simulink model "__AAVAvionics"  (Simulink 6.0)
settings: Solver=ode45  StartTime=0.0  StopTime=10.0  RelTol=1e-3
settings Model: LastModifiedBy=root

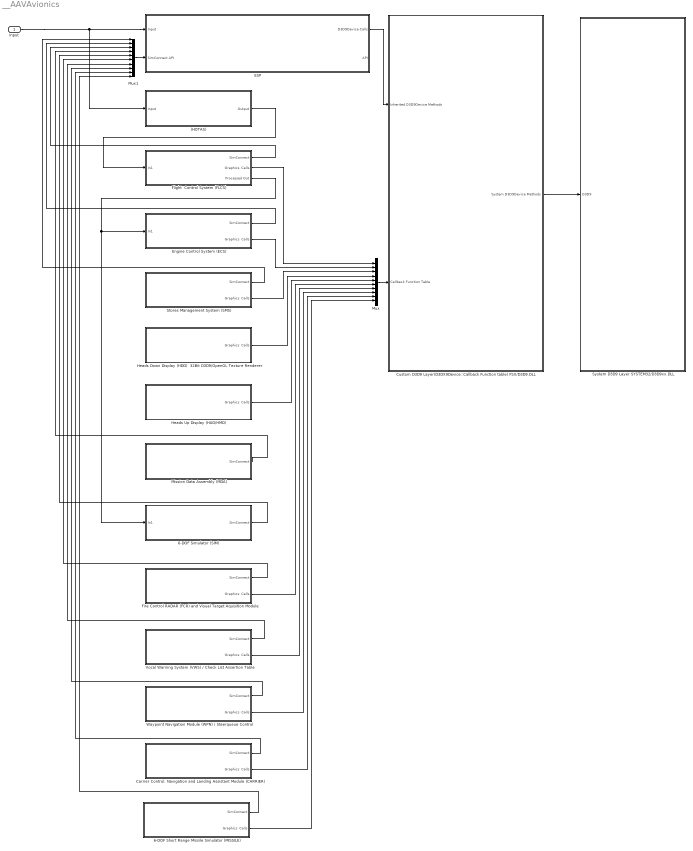
== system __AAVAvionics ==
  Input : Inport  Port=1  LatchInput=off
  (HOTAS) : Subsystem
  6-DOF Short Range Missile Simulator (MISSILE) : Subsystem
  6-DOF Simulator (SIM) : Subsystem
  "Carrier Control, Navigation and Landing Assistant Module (CARRIER)" : Subsystem
  Custom D3D9 Layer(D3DX9Device::Callback Function table) FSX/D3D9.DLL : Subsystem
  ESP : Subsystem
  Engine Control System (ECS) : Subsystem
  Fire Control RADAR (FCR) and Visual Target Aquisition Module : Subsystem
  Flight  Control System (FLCS) : Subsystem
  Heads Down Display (HDD)  32Bit D3D9/OpenGL Texture Renderer : Subsystem
  Heads Up Display (HUD/HMD) : Subsystem
  Mission Data Assembly (MDA) : Subsystem
  Mux : Mux  Inputs=10
  Mux1 : Mux  Inputs=10
  Stores Management System (SMS) : Subsystem
  System D3D9 Layer SYSTEM32/D3D9xx.DLL : Subsystem
  "Vocal Warning System (VWS) / Check List Assertion Table " : Subsystem
  Waypoint Navigation Module (WPN) / Steerqueue Control : Subsystem
  wires:
  ESP/1("D3D9Device Calls ") -> Custom D3D9 Layer(D3DX9Device::Callback Function table) FSX/D3D9.DLL/1(Inherited D3D9Device Methods)
  Custom D3D9 Layer(D3DX9Device::Callback Function table) FSX/D3D9.DLL/1(System D3D9Device Methods) -> System D3D9 Layer SYSTEM32/D3D9xx.DLL/1(D3D9)
  Input/1 -> ESP/1(Input), (HOTAS)/1(Input)
  Mux/1 -> Custom D3D9 Layer(D3DX9Device::Callback Function table) FSX/D3D9.DLL/2(Callback Function Table)
  Engine Control System (ECS)/2(Graphics  Calls) -> Mux/2
  (HOTAS)/1(Output) -> Flight  Control System (FLCS)/1(In1)
  Flight  Control System (FLCS)/2(Graphics  Calls) -> Mux/1
  Flight  Control System (FLCS)/3(Processed Out) -> Engine Control System (ECS)/1(In1), 6-DOF Simulator (SIM)/1(In1)
  Stores Management System (SMS)/2(Graphics  Calls) -> Mux/3
  Stores Management System (SMS)/1(SimConnect) -> Mux1/1
  Mux1/1 -> ESP/2(SimConnect API)
  Flight  Control System (FLCS)/1(SimConnect) -> Mux1/3
  Engine Control System (ECS)/1(SimConnect) -> Mux1/2
  Heads Down Display (HDD)  32Bit D3D9/OpenGL Texture Renderer/1(Graphics  Calls) -> Mux/4
  Heads Up Display (HUD/HMD)/1(Graphics  Calls) -> Mux/5
  Mission Data Assembly (MDA)/1(SimConnect) -> Mux1/4
  6-DOF Simulator (SIM)/1(SimConnect) -> Mux1/5
  Fire Control RADAR (FCR) and Visual Target Aquisition Module/2(Graphics  Calls) -> Mux/6
  Fire Control RADAR (FCR) and Visual Target Aquisition Module/1(SimConnect) -> Mux1/6
  "Vocal Warning System (VWS) / Check List Assertion Table "/2(Graphics  Calls) -> Mux/7
  Waypoint Navigation Module (WPN) / Steerqueue Control/2(Graphics  Calls) -> Mux/8
  "Vocal Warning System (VWS) / Check List Assertion Table "/1(SimConnect) -> Mux1/7
  Waypoint Navigation Module (WPN) / Steerqueue Control/1(SimConnect) -> Mux1/8
  "Carrier Control, Navigation and Landing Assistant Module (CARRIER)"/2(Graphics  Calls) -> Mux/9
  "Carrier Control, Navigation and Landing Assistant Module (CARRIER)"/1(SimConnect) -> Mux1/9
  6-DOF Short Range Missile Simulator (MISSILE)/1(SimConnect) -> Mux1/10
  6-DOF Short Range Missile Simulator (MISSILE)/2(Graphics  Calls) -> Mux/10

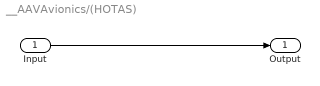
== system __AAVAvionics/(HOTAS) ==
  Input : Inport  Port=1  LatchInput=off
  Output : Outport
  wires:
  Input/1 -> Output/1

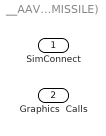
== system __AAVAvionics/6-DOF Short Range Missile Simulator (MISSILE) ==
  SimConnect : Outport
  Graphics  Calls : Outport  Port=2

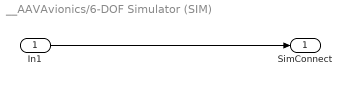
== system __AAVAvionics/6-DOF Simulator (SIM) ==
  In1 : Inport  Port=1  LatchInput=off
  SimConnect : Outport
  wires:
  In1/1 -> SimConnect/1

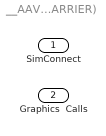
== system __AAVAvionics/Carrier Control, Navigation and Landing Assistant Module (CARRIER) ==
  SimConnect : Outport
  Graphics  Calls : Outport  Port=2

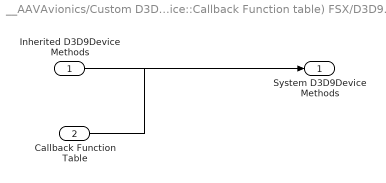
== system __AAVAvionics/Custom D3D9 Layer(D3DX9Device::Callback Function table) FSX/D3D9.DLL ==
  Inherited D3D9Device Methods : Inport  Port=1  LatchInput=off
  Callback Function Table : Inport  Port=2  LatchInput=off
  System D3D9Device Methods : Outport
  wires:
  Inherited D3D9Device Methods/1 -> System D3D9Device Methods/1
  Callback Function Table/1 -> ?

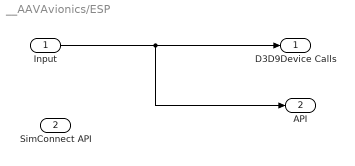
== system __AAVAvionics/ESP ==
  Input : Inport  Port=1  LatchInput=off
  SimConnect API : Inport  Port=2  LatchInput=off
  "D3D9Device Calls " : Outport
  API : Outport  Port=2
  wires:
  Input/1 -> "D3D9Device Calls "/1, API/1

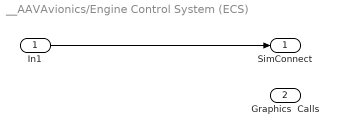
== system __AAVAvionics/Engine Control System (ECS) ==
  In1 : Inport  Port=1  LatchInput=off
  SimConnect : Outport
  Graphics  Calls : Outport  Port=2
  wires:
  In1/1 -> SimConnect/1

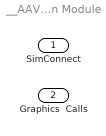
== system __AAVAvionics/Fire Control RADAR (FCR) and Visual Target Aquisition Module ==
  SimConnect : Outport
  Graphics  Calls : Outport  Port=2

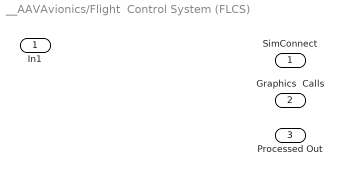
== system __AAVAvionics/Flight  Control System (FLCS) ==
  In1 : Inport  Port=1  LatchInput=off
  SimConnect : Outport
  Graphics  Calls : Outport  Port=2
  Processed Out : Outport  Port=3

== system __AAVAvionics/Heads Down Display (HDD)  32Bit D3D9/OpenGL Texture Renderer ==
  Graphics  Calls : Outport

== system __AAVAvionics/Heads Up Display (HUD/HMD) ==
  Graphics  Calls : Outport

== system __AAVAvionics/Mission Data Assembly (MDA) ==
  SimConnect : Outport

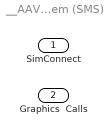
== system __AAVAvionics/Stores Management System (SMS) ==
  SimConnect : Outport
  Graphics  Calls : Outport  Port=2

== system __AAVAvionics/System D3D9 Layer SYSTEM32/D3D9xx.DLL ==
  D3D9 : Inport  Port=1  LatchInput=off

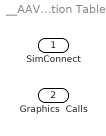
== system __AAVAvionics/Vocal Warning System (VWS) / Check List Assertion Table  ==
  SimConnect : Outport
  Graphics  Calls : Outport  Port=2

== system __AAVAvionics/Waypoint Navigation Module (WPN) / Steerqueue Control ==
  SimConnect : Outport
  Graphics  Calls : Outport  Port=2
